simulink model "TinBotPhysical"  (Simulink 8.7)
settings: Solver=VariableStepAuto  StartTime=0.0  StopTime=10.0  RelTol=1e-3
settings Model: Creator=maximilian  LastModifiedBy=maximilian
settings DataIOCC: LimitDataPoints=off  SaveFormat=Dataset
settings DebuggingCC: UnderspecifiedInitializationDetection=Simplified  MergeDetectMultiDrivingBlocksExec=error
settings HardwareCC: ProdBitPerPointer=64  ProdLargestAtomicFloat=Float  ProdIntDivRoundTo=Zero  ProdEndianess=LittleEndian  ProdWordSize=64  ProdHWDeviceType=Intel->x86-64 (Windows64)
settings ModelReferenceCC: PropagateSignalLabelsOutOfModel=on
settings ConfigComp: CovModelRefEnable=off

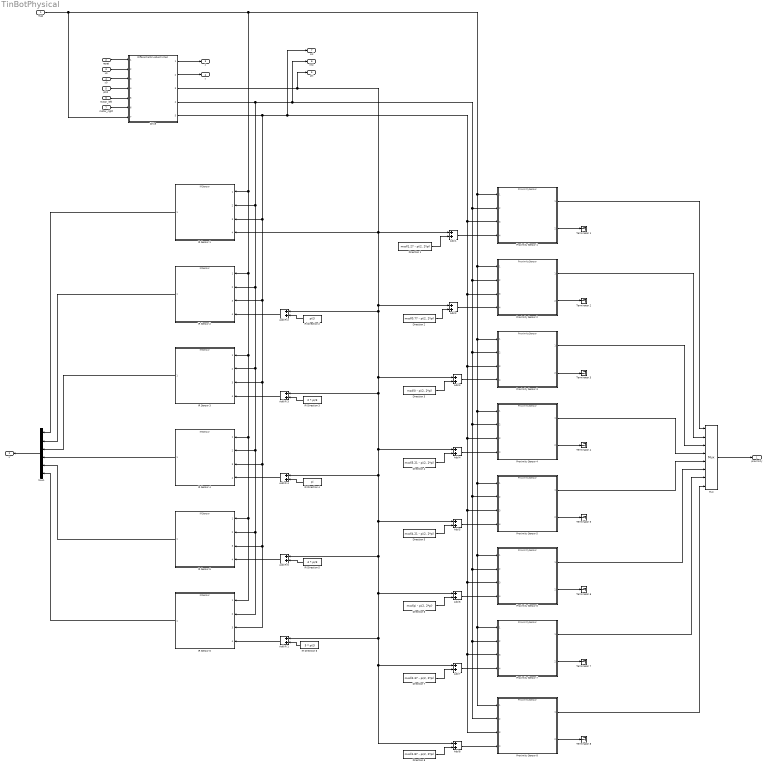
== system TinBotPhysical ==
  map : Inport
  reset : Inport  Port=2
  x0 : Inport  Port=3
  y0 : Inport  Port=4
  phi0 : Inport  Port=5
  motor_left : Inport  Port=6
  motor_right : Inport  Port=7
  Add {1..8} (8 alike) : Sum
  Add IR {1..5} (5 alike) : Sum
  Direction 1 : Constant  Value=mod(1.27 - pi/2, 2*pi)
  Direction 2 : Constant  Value=mod(0.77 - pi/2, 2*pi)
  Direction 3 : Constant  Value=mod(0 - pi/2, 2*pi)
  Direction 4 : Constant  Value=mod(5.21 - pi/2, 2*pi)
  Direction 5 : Constant  Value=mod(4.21 - pi/2, 2*pi)
  Direction 6 : Constant  Value=mod(pi - pi/2, 2*pi)
  Direction 7 : Constant  Value=mod(2.37 - pi/2, 2*pi)
  Direction 8 : Constant  Value=mod(1.87 - pi/2, 2*pi)
  Drive : ModelReference  ModelNameDialog=DifferentialDriveRestricted.mdl  SimulationMode=Normal  ModelReferenceVersion=1.40
  IR Direction 2 : Constant  Value=pi/3
  IR Direction 3 : Constant  Value=2 * pi/3
  IR Direction 4 : Constant  Value=pi
  IR Direction 5 : Constant  Value=4 * pi/3
  IR Direction 6 : Constant  Value=5 * pi/3
  IR Sensor {1..6} (6 alike) : ModelReference  ModelNameDialog=IRSensor.mdl  SimulationMode=Normal  ModelReferenceVersion=1.7
  Mux : Mux  Inputs=8
  Mux1 : Mux  Inputs=6
  Proximity Sensor {1..8} (8 alike) : ModelReference  ModelNameDialog=ProximitySensor.mdl  SimulationMode=Normal  ModelReferenceVersion=1.12
  Terminator {1..8} (8 alike) : Terminator
  proximity : Outport  PortDimensions=8
  ir : Outport  Port=2
  x : Outport  Port=3
  y : Outport  Port=4
  phi : Outport  Port=5
  row : Outport  Port=6
  col : Outport  Port=7
  wires:
  map/1 -> Drive/7, Proximity Sensor 4/1, Proximity Sensor 5/1, Proximity Sensor 6/1, Proximity Sensor 7/1, Proximity Sensor 8/1, Proximity Sensor 3/1, Proximity Sensor 2/1, Proximity Sensor 1/1, IR Sensor 1/1, IR Sensor 6/1, IR Sensor 5/1, IR Sensor 4/1, IR Sensor 3/1, IR Sensor 2/1
  Add 1/1 -> Proximity Sensor 1/4
  Direction 1/1 -> Add 1/2
  Add 2/1 -> Proximity Sensor 2/4
  Direction 2/1 -> Add 2/2
  Add 3/1 -> Proximity Sensor 3/4
  Direction 3/1 -> Add 3/2
  Add 4/1 -> Proximity Sensor 4/4
  Direction 4/1 -> Add 4/2
  Add 5/1 -> Proximity Sensor 5/4
  Direction 5/1 -> Add 5/2
  Add 6/1 -> Proximity Sensor 6/4
  Direction 6/1 -> Add 6/2
  Add 7/1 -> Proximity Sensor 7/4
  Direction 7/1 -> Add 7/2
  Add 8/1 -> Proximity Sensor 8/4
  Direction 8/1 -> Add 8/2
  Drive/4 -> row/1, Proximity Sensor 8/2, Proximity Sensor 7/2, Proximity Sensor 6/2, Proximity Sensor 5/2, Proximity Sensor 4/2, Proximity Sensor 3/2, Proximity Sensor 2/2, Proximity Sensor 1/2, IR Sensor 6/2, IR Sensor 5/2, IR Sensor 4/2, IR Sensor 3/2, IR Sensor 2/2, IR Sensor 1/2
  Proximity Sensor 1/1 -> Mux/1
  Proximity Sensor 2/1 -> Mux/2
  Proximity Sensor 3/1 -> Mux/3
  Proximity Sensor 4/1 -> Mux/4
  Proximity Sensor 5/1 -> Mux/5
  Proximity Sensor 6/1 -> Mux/6
  Proximity Sensor 7/1 -> Mux/7
  Proximity Sensor 8/1 -> Mux/8
  Mux/1 -> proximity/1
  Drive/3 -> phi/1, Add 8/1, Add 7/1, Add IR 1/1, Add 6/1, Add IR 5/1, Add 5/1, Add IR 4/1, Add 4/1, Add IR 3/1, Add 3/1, Add IR 2/1, Add 2/1, IR Sensor 1/4, Add 1/1
  Add IR 2/1 -> IR Sensor 2/4
  IR Direction 2/1 -> Add IR 2/2
  IR Direction 3/1 -> Add IR 3/2
  Add IR 3/1 -> IR Sensor 3/4
  IR Direction 4/1 -> Add IR 4/2
  Add IR 4/1 -> IR Sensor 4/4
  Add IR 5/1 -> IR Sensor 5/4
  IR Direction 5/1 -> Add IR 5/2
  Add IR 1/1 -> IR Sensor 6/4
  IR Direction 6/1 -> Add IR 1/2
  IR Sensor 1/1 -> Mux1/1
  IR Sensor 2/1 -> Mux1/2
  IR Sensor 3/1 -> Mux1/3
  IR Sensor 4/1 -> Mux1/4
  IR Sensor 5/1 -> Mux1/5
  IR Sensor 6/1 -> Mux1/6
  Mux1/1 -> ir/1
  Proximity Sensor 5/2 -> Terminator 5/1
  Proximity Sensor 6/2 -> Terminator 6/1
  Proximity Sensor 4/2 -> Terminator 4/1
  Proximity Sensor 3/2 -> Terminator 3/1
  Proximity Sensor 2/2 -> Terminator 2/1
  Proximity Sensor 1/2 -> Terminator 1/1
  Proximity Sensor 7/2 -> Terminator 7/1
  Proximity Sensor 8/2 -> Terminator 8/1
  Drive/1 -> x/1
  Drive/2 -> y/1
  Drive/5 -> IR Sensor 6/3, IR Sensor 5/3, IR Sensor 4/3, IR Sensor 3/3, IR Sensor 2/3, IR Sensor 1/3, col/1, Proximity Sensor 8/3, Proximity Sensor 7/3, Proximity Sensor 6/3, Proximity Sensor 5/3, Proximity Sensor 4/3, Proximity Sensor 3/3, Proximity Sensor 2/3, Proximity Sensor 1/3
  reset/1 -> Drive/1
  x0/1 -> Drive/2
  y0/1 -> Drive/3
  phi0/1 -> Drive/4
  motor_left/1 -> Drive/5
  motor_right/1 -> Drive/6
